simulink model "Clark"  (R2014b)
settings: Solver=ode45  StartTime=0.0  StopTime=0.2  RelTol=1e-3
settings Model: Creator=Lei  LastModifiedBy=Lei

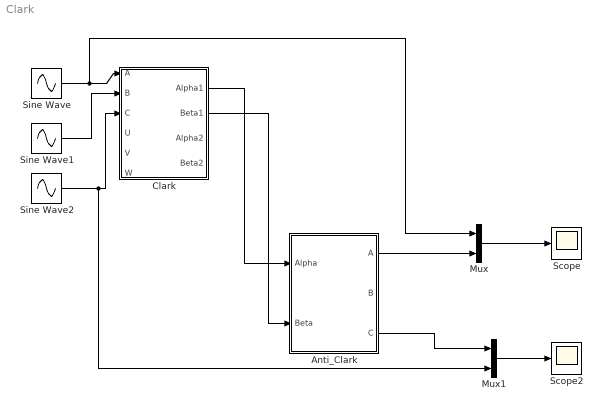
== system Clark ==
  Anti_Clark : Subsystem
  Clark : Subsystem
  Mux : Mux  Inputs=2
  Mux1 : Mux  Inputs=2
  Scope : Scope
      settings: YMin=-150  YMax=150
  Scope2 : Scope
      settings: YMin=-150  YMax=150  SaveName=ScopeData2
  Sine Wave : Sin  Amplitude=100  Frequency=2*pi*50  SampleTime=10e-6
  Sine Wave1 : Sin  Amplitude=100  Frequency=2*pi*50  Phase=-2/3*pi  SampleTime=10e-6
  Sine Wave2 : Sin  Amplitude=100  Frequency=2*pi*50  Phase=2/3*pi  SampleTime=10e-6
  wires:
  Sine Wave1/1 -> Clark/2(B)
  Sine Wave2/1 -> Mux1/2, Clark/3(C)
  Clark/2(Beta1) -> Anti_Clark/2(Beta)
  Clark/1(Alpha1) -> Anti_Clark/1(Alpha)
  Anti_Clark/3(C) -> Mux1/1
  Anti_Clark/1(A) -> Mux/2
  Sine Wave/1 -> Mux/1, Clark/1(A)
  Mux/1 -> Scope/1
  Mux1/1 -> Scope2/1

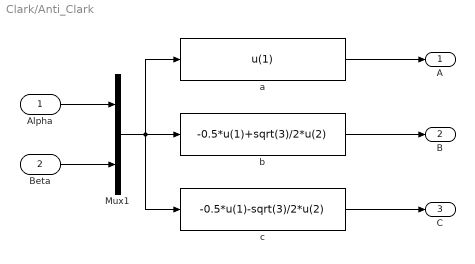
== system Clark/Anti_Clark ==
  Alpha : Inport
  Beta : Inport  Port=2
  Mux1 : Mux  Inputs=2
  a : Fcn  Expr=u(1)
  b : Fcn  Expr=-0.5*u(1)+sqrt(3)/2*u(2)
  c : Fcn  Expr=-0.5*u(1)-sqrt(3)/2*u(2)
  A : Outport
  B : Outport  Port=2
  C : Outport  Port=3
  wires:
  b/1 -> B/1
  c/1 -> C/1
  Beta/1 -> Mux1/2
  Alpha/1 -> Mux1/1
  a/1 -> A/1
  Mux1/1 -> a/1, c/1, b/1

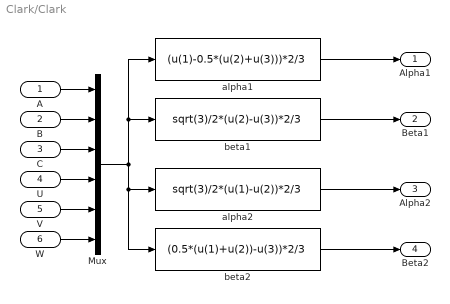
== system Clark/Clark ==
  A : Inport
  B : Inport  Port=2
  C : Inport  Port=3
  U : Inport  Port=4
  V : Inport  Port=5
  W : Inport  Port=6
  Mux : Mux  Inputs=6
  alpha1 : Fcn  Expr=(u(1)-0.5*(u(2)+u(3)))*2/3
  alpha2 : Fcn  Expr=sqrt(3)/2*(u(1)-u(2))*2/3
  beta1 : Fcn  Expr=sqrt(3)/2*(u(2)-u(3))*2/3
  beta2 : Fcn  Expr=(0.5*(u(1)+u(2))-u(3))*2/3
  Alpha1 : Outport
  Beta1 : Outport  Port=2
  Alpha2 : Outport  Port=3
  Beta2 : Outport  Port=4
  wires:
  alpha1/1 -> Alpha1/1
  B/1 -> Mux/2
  C/1 -> Mux/3
  A/1 -> Mux/1
  beta1/1 -> Beta1/1
  U/1 -> Mux/4
  V/1 -> Mux/5
  W/1 -> Mux/6
  alpha2/1 -> Alpha2/1
  beta2/1 -> Beta2/1
  Mux/1 -> alpha2/1, beta2/1, beta1/1, alpha1/1
